simulink library "perturbations"  (R2025b)
settings: Solver=VariableStepAuto  StartTime=0.0  StopTime=10.0  RelTol=1e-3
values from neighbouring files (symbols this model uses):
  e_sun = deg2rad(23.45)    [project_review.m]
  I = diag([ix iy iz])    [project_review.m]
  j = [0.01; 0.05; 0.01;]    [project_review.m]
  mu_E = G_E*M_E    (= 398199)    [project_review.m]
  n_sun = 2*pi / T_sun    (= 1.99102127766e-07)    [project_review.m]
  R_E = 6378    [project_review.m]
  sim_step = 0.01    [project_review.m]
  w_E = 7.27 * 10^-5    (= 7.27e-05)    [project_review.m]
undefined symbols (not defined in the file or in its folder): area, g_10, g_11, h_11, N_B, P, r_Fi, r_sun, rho_d, rho_s
libraries: matrix_library x4, vec_norm x3
settings Model: Creator=nicol  LastModifiedBy=nicol

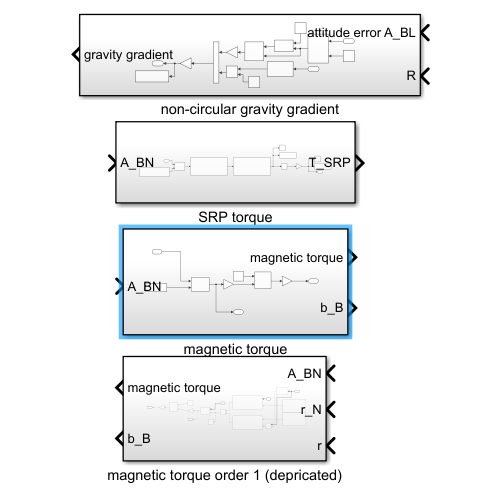
[thumbnail: Simulink's stored preview of the top-level diagram]
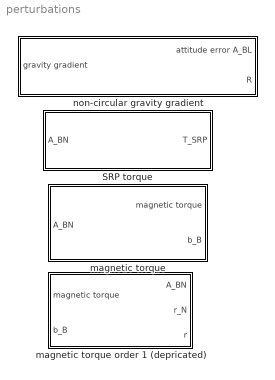
== system perturbations ==
  SRP torque : Subsystem
  magnetic torque : Subsystem
  magnetic torque order 1 (depricated) : Subsystem
  non-circular gravity gradient : Subsystem
      settings: PortSchema="{\"entries\":[{\"content\":{\"sides\":[{\"content\":{\"connectorIds\":[\"Out1\"]},\"type\":\"ConnectorPlacement.EquallySpacedRectSide\",\"uuid\":\"2a67419a-68c9-4369-a698-e6ac26417455\"},{\"content\":{\"connectorIds\":[\"In1\",\"In2\"],\"side\":\"RIGHT\"},\"type\":\"ConnectorPlacement.EquallySpacedRectSide\",\"uuid\":\"5f3f4c4a-6b79-4b92-8f4c-19ffa36753b2\"},{\"content\":{\"side\":\"TOP\"},\"type\":\"ConnectorPlacement.EquallySpacedRectSide\",\"uuid\":\"22c946b7-ea77-4444-a63c-d5b3d585f671\"}]},\"type\":\"ConnectorPlacement.EquallySpacedConnector\",\"uuid\":\"037c4a72-b28b-418e-a921-9da68dc0cd93\"}],\"packageUris\":[\"http://schema.mathworks.com/mf0/Connector/R2020b\"],\"version\":\"1.0\"}"

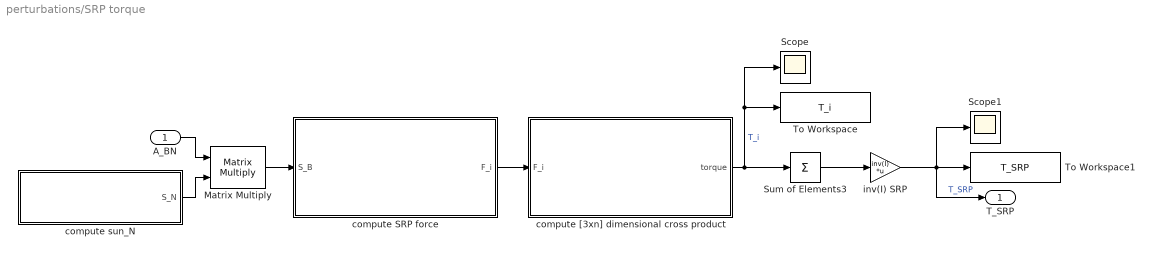
== system perturbations/SRP torque ==
  A_BN : Inport
  Matrix Multiply : Product  Multiplication=Matrix(*)
  Scope : Scope
      settings: ActiveDisplayYMinimum=-1  ActiveDisplayYMaximum=1  DataLoggingVariableName=ScopeData6
  Scope1 : Scope
      settings: ActiveDisplayYMinimum=-7.5910805781117744E-24  ActiveDisplayYMaximum=7.5910805781117744E-24  DataLoggingVariableName=ScopeData7
  Sum of Elements3 : Sum  Inputs=+  CollapseMode=Specified dimension  CollapseDim=2
  To Workspace : ToWorkspace  VariableName=T_i  SaveFormat=Timeseries  SampleTime=-1
  To Workspace1 : ToWorkspace  VariableName=T_SRP  SaveFormat=Timeseries  SampleTime=-1
  compute SRP force : Subsystem
  compute [3xn] dimensional cross product : Subsystem
  compute sun_N : Subsystem
  inv(I) SRP : Gain  Gain=inv(I)  Multiplication=Matrix(K*u)
  T_SRP : Outport
  wires:
  compute [3xn] dimensional cross product/1(torque) -> To Workspace/1, Scope/1, Sum of Elements3/1  "T_i"
  compute SRP force/1(F_i) -> compute [3xn] dimensional cross product/1(F_i)
  Matrix Multiply/1 -> compute SRP force/1(S_B)
  compute sun_N/1(S_N) -> Matrix Multiply/2
  inv(I) SRP/1 -> Scope1/1, T_SRP/1, To Workspace1/1  "T_SRP"
  A_BN/1 -> Matrix Multiply/1
  Sum of Elements3/1 -> inv(I) SRP/1

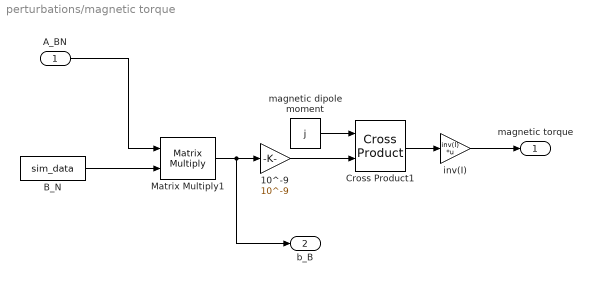
== system perturbations/magnetic torque ==
  A_BN : Inport
  10^-9 : Gain  Gain=10^-9
  B_N : FromWorkspace  VariableName=sim_data  SampleTime=sim_step  Interpolate=off  OutputAfterFinalValue=Holding final value
  Cross Product1 : matrix_library/Cross Product
  Matrix Multiply1 : Product  Multiplication=Matrix(*)
  inv(I) : Gain  Gain=inv(I)  Multiplication=Matrix(K*u)
  magnetic dipole moment : Constant  Value=j
  magnetic torque : Outport
  b_B : Outport  Port=2
  wires:
  A_BN/1 -> Matrix Multiply1/1
  magnetic dipole moment/1 -> Cross Product1/1
  B_N/1 -> Matrix Multiply1/2
  Cross Product1/1 -> inv(I)/1
  inv(I)/1 -> magnetic torque/1
  Matrix Multiply1/1 -> b_B/1, 10^-9/1
  10^-9/1 -> Cross Product1/2

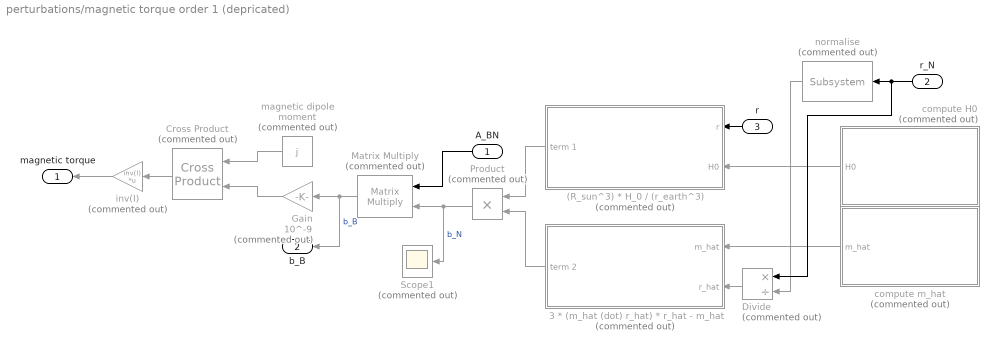
== system perturbations/magnetic torque order 1 (depricated) ==
  A_BN : Inport
  r_N : Inport  Port=2
  r : Inport  Port=3
  (R_sun^3) * H_0 / (r_earth^3) : Subsystem  Commented=on
      settings: PortSchema="{\"entries\":[{\"content\":{\"sides\":[{\"content\":{\"connectorIds\":[\"Out1\"]},\"type\":\"ConnectorPlacement.EquallySpacedRectSide\",\"uuid\":\"bbe988fc-17c4-4719-9870-44bc4a4e76ce\"},{\"content\":{\"connectorIds\":[\"In1\",\"In2\"],\"side\":\"RIGHT\"},\"type\":\"ConnectorPlacement.EquallySpacedRectSide\",\"uuid\":\"575c26dc-e0b7-4e24-b262-40ca05ffcfe5\"},{\"content\":{\"side\":\"TOP\"},\"type\":\"ConnectorPlacement.EquallySpacedRectSide\",\"uuid\":\"0bdf66e4-cddb-4706-9c0a-b23684b15a0a\"}]},\"type\":\"ConnectorPlacement.EquallySpacedConnector\",\"uuid\":\"a70c04a6-2589-454e-b011-fc54f6acc766\"}],\"packageUris\":[\"http://schema.mathworks.com/mf0/Connector/R2020b\"],\"version\":\"1.0\"}"
  3 * (m_hat (dot) r_hat) * r_hat - m_hat : Subsystem  Commented=on
  Cross Product : matrix_library/Cross Product  Commented=on
  Divide : Product  Commented=on  Inputs=*/
  Gain : Gain  Commented=on  Gain=10^-9
  Matrix Multiply : Product  Commented=on  Multiplication=Matrix(*)
  Product : Product  Commented=on
  Scope1 : Scope  Commented=on
      settings: DataLoggingVariableName=ScopeData2
  compute H0 : Subsystem  Commented=on
      settings: PortSchema="{\"entries\":[{\"content\":{\"sides\":[{\"content\":{\"connectorIds\":[\"Out1\"]},\"type\":\"ConnectorPlacement.EquallySpacedRectSide\",\"uuid\":\"69538ac4-798d-499e-8a01-9dbb1ae91e13\"},{\"content\":{\"side\":\"RIGHT\"},\"type\":\"ConnectorPlacement.EquallySpacedRectSide\",\"uuid\":\"e472a16b-e756-43b0-a684-24a7beecf6b1\"},{\"content\":{\"side\":\"TOP\"},\"type\":\"ConnectorPlacement.EquallySpacedRectSide\",\"uuid\":\"c0da2b73-1d3e-4f5f-b1be-bce0e733f90d\"}]},\"type\":\"ConnectorPlacement.EquallySpacedConnector\",\"uuid\":\"edf54bcc-843b-4ee1-a337-02c9fdc591b1\"}],\"packageUris\":[\"http://schema.mathworks.com/mf0/Connector/R2020b\"],\"version\":\"1.0\"}"
  compute m_hat : Subsystem  Commented=on
      settings: PortSchema="{\"entries\":[{\"content\":{\"sides\":[{\"content\":{\"connectorIds\":[\"Out1\"]},\"type\":\"ConnectorPlacement.EquallySpacedRectSide\",\"uuid\":\"69538ac4-798d-499e-8a01-9dbb1ae91e13\"},{\"content\":{\"side\":\"RIGHT\"},\"type\":\"ConnectorPlacement.EquallySpacedRectSide\",\"uuid\":\"e472a16b-e756-43b0-a684-24a7beecf6b1\"},{\"content\":{\"side\":\"TOP\"},\"type\":\"ConnectorPlacement.EquallySpacedRectSide\",\"uuid\":\"c0da2b73-1d3e-4f5f-b1be-bce0e733f90d\"}]},\"type\":\"ConnectorPlacement.EquallySpacedConnector\",\"uuid\":\"edf54bcc-843b-4ee1-a337-02c9fdc591b1\"}],\"packageUris\":[\"http://schema.mathworks.com/mf0/Connector/R2020b\"],\"version\":\"1.0\"}"
  inv(I) : Gain  Commented=on  Gain=inv(I)  Multiplication=Matrix(K*u)
  magnetic dipole moment : Constant  Commented=on  Value=j
  normalise : vec_norm/Subsystem  Commented=on  SystemSampleTime=-1  VariantActivationTime=update diagram  EmptyChoice=off  PassThrough=off  PassThroughVariantControl=(default)  EmptyChoiceVariantControl=(default)  AllowFlexibleInterface=on  Latency=0  AutoFrameSizeCalculation=off
  magnetic torque : Outport
  b_B : Outport  Port=2
  wires:
  A_BN/1 -> Matrix Multiply/1
  inv(I)/1 -> magnetic torque/1
  3 * (m_hat (dot) r_hat) * r_hat - m_hat/1(term 2) -> Product/2
  (R_sun^3) * H_0 / (r_earth^3)/1(term 1) -> Product/1
  compute m_hat/1(m_hat) -> 3 * (m_hat (dot) r_hat) * r_hat - m_hat/1(m_hat)
  magnetic dipole moment/1 -> Cross Product/1
  Product/1 -> Scope1/1, Matrix Multiply/2  "b_N"
  Matrix Multiply/1 -> b_B/1, Gain/1  "b_B"
  compute H0/1(H0) -> (R_sun^3) * H_0 / (r_earth^3)/2(H0)
  Divide/1 -> 3 * (m_hat (dot) r_hat) * r_hat - m_hat/2(r_hat)
  normalise/1 -> Divide/2
  r_N/1 -> normalise/1, Divide/1
  Cross Product/1 -> inv(I)/1
  Gain/1 -> Cross Product/2
  r/1 -> (R_sun^3) * H_0 / (r_earth^3)/1(r)

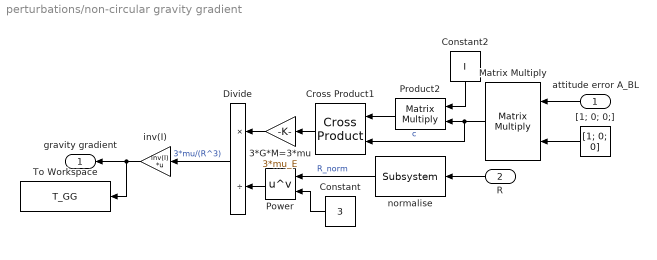
== system perturbations/non-circular gravity gradient ==
  attitude error A_BL : Inport
  R : Inport  Port=2
  3*G*M=3*mu : Gain  Gain=3*mu_E
  Constant : Constant  Value=3
  Constant2 : Constant  Value=I
  Cross Product1 : matrix_library/Cross Product
  Divide : Product  Inputs=*/
  Matrix Multiply : Product  Multiplication=Matrix(*)
  Power : Math  Operator=pow
  Product2 : Product  Multiplication=Matrix(*)
  To Workspace : ToWorkspace  VariableName=T_GG  SaveFormat=Timeseries  SampleTime=-1
  "[1; 0; 0;]" : Constant  Value=[1; 0; 0]
  inv(I) : Gain  Gain=inv(I)  Multiplication=Matrix(K*u)
  normalise : vec_norm/Subsystem  SystemSampleTime=-1  VariantActivationTime=update diagram  EmptyChoice=off  PassThrough=off  PassThroughVariantControl=(default)  EmptyChoiceVariantControl=(default)  AllowFlexibleInterface=on  Latency=0  AutoFrameSizeCalculation=off
  gravity gradient : Outport
  wires:
  normalise/1 -> Power/1  "R_norm"
  Power/1 -> Divide/2
  Constant/1 -> Power/2
  R/1 -> normalise/1
  inv(I)/1 -> To Workspace/1, gravity gradient/1
  3*G*M=3*mu/1 -> Divide/1
  "[1; 0; 0;]"/1 -> Matrix Multiply/2
  Product2/1 -> Cross Product1/1
  Cross Product1/1 -> 3*G*M=3*mu/1
  Constant2/1 -> Product2/1
  attitude error A_BL/1 -> Matrix Multiply/1
  Matrix Multiply/1 -> Product2/2, Cross Product1/2  "c"
  Divide/1 -> inv(I)/1  "3*mu/(R^3)"

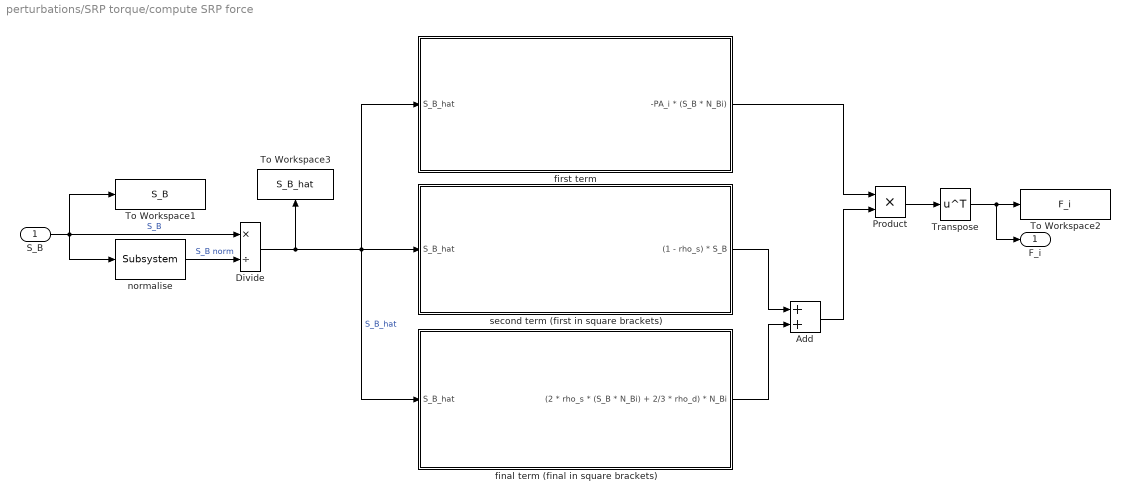
== system perturbations/SRP torque/compute SRP force ==
  S_B : Inport
  Add : Sum
  Divide : Product  Inputs=*/
  Product : Product
  To Workspace1 : ToWorkspace  VariableName=S_B  SaveFormat=Timeseries  SampleTime=-1
  To Workspace2 : ToWorkspace  VariableName=F_i  SaveFormat=Timeseries  SampleTime=-1
  To Workspace3 : ToWorkspace  VariableName=S_B_hat  SaveFormat=Timeseries  SampleTime=-1
  Transpose : Math  Operator=transpose
  final term (final in square brackets) : Subsystem
  first term : Subsystem
  normalise : vec_norm/Subsystem  SystemSampleTime=-1  VariantActivationTime=update diagram  EmptyChoice=off  PassThrough=off  PassThroughVariantControl=(default)  EmptyChoiceVariantControl=(default)  AllowFlexibleInterface=on  Latency=0  AutoFrameSizeCalculation=off
  second term (first in square brackets) : Subsystem
  F_i : Outport
  wires:
  final term (final in square brackets)/1((2 * rho_s * (S_B * N_Bi) + 2/3 * rho_d) * N_Bi) -> Add/2
  Transpose/1 -> F_i/1, To Workspace2/1
  first term/1(-PA_i * (S_B * N_Bi)) -> Product/1
  Add/1 -> Product/2
  second term (first in square brackets)/1((1 - rho_s) * S_B) -> Add/1
  Product/1 -> Transpose/1
  normalise/1 -> Divide/2  "S_B norm"
  Divide/1 -> second term (first in square brackets)/1(S_B_hat), first term/1(S_B_hat), final term (final in square brackets)/1(S_B_hat), To Workspace3/1  "S_B_hat"
  S_B/1 -> normalise/1, Divide/1, To Workspace1/1  "S_B"

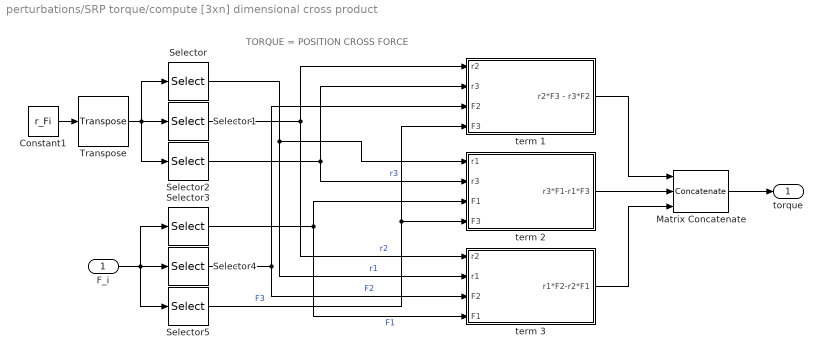
== system perturbations/SRP torque/compute [3xn] dimensional cross product ==
  note: TORQUE = POSITION CROSS FORCE
  F_i : Inport
  Constant1 : Constant  Value=r_Fi
  Matrix Concatenate : Concatenate  NumInputs=3  Mode=Multidimensional array
  Selector : Selector  NumberOfDimensions=2  InputPortWidth=3  IndexOptions=Index vector (dialog),Select all  Indices=1,1  OutputSizes=1,1
  Selector1 : Selector  NumberOfDimensions=2  InputPortWidth=3  IndexOptions=Index vector (dialog),Select all  Indices=2,1  OutputSizes=1,1
  Selector2 : Selector  NumberOfDimensions=2  InputPortWidth=3  IndexOptions=Index vector (dialog),Select all  Indices=3,1  OutputSizes=1,1
  Selector3 : Selector  NumberOfDimensions=2  InputPortWidth=3  IndexOptions=Index vector (dialog),Select all  Indices=1,1  OutputSizes=1,1
  Selector4 : Selector  NumberOfDimensions=2  InputPortWidth=3  IndexOptions=Index vector (dialog),Select all  Indices=2,1  OutputSizes=1,1
  Selector5 : Selector  NumberOfDimensions=2  InputPortWidth=3  IndexOptions=Index vector (dialog),Select all  Indices=3,1  OutputSizes=1,1
  Transpose : matrix_library/Transpose
  term 1 : Subsystem
  term 2 : Subsystem
  term 3 : Subsystem
  torque : Outport
  wires:
  Constant1/1 -> Transpose/1
  F_i/1 -> Selector4/1, Selector3/1, Selector5/1
  term 2/1(r3*F1-r1*F3) -> Matrix Concatenate/2
  Selector1/1 -> term 1/1(r2), term 3/1(r2)  "r2"
  term 3/1(r1*F2-r2*F1) -> Matrix Concatenate/3
  term 1/1(r2*F3 - r3*F2) -> Matrix Concatenate/1
  Selector4/1 -> term 3/3(F2), term 1/3(F2)  "F2"
  Selector5/1 -> term 1/4(F3), term 2/4(F3)  "F3"
  Selector2/1 -> term 1/2(r3), term 2/2(r3)  "r3"
  Transpose/1 -> Selector1/1, Selector/1, Selector2/1
  Selector3/1 -> term 3/4(F1), term 2/3(F1)  "F1"
  Selector/1 -> term 3/2(r1), term 2/1(r1)  "r1"
  Matrix Concatenate/1 -> torque/1

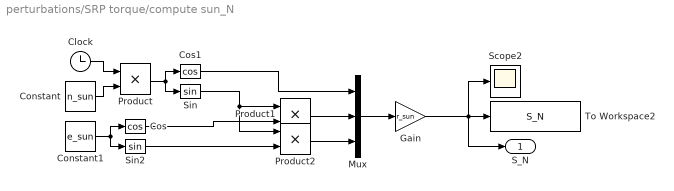
== system perturbations/SRP torque/compute sun_N ==
  Clock : Clock
  Constant : Constant  Value=n_sun
  Constant1 : Constant  Value=e_sun
  Cos : Trigonometry  Operator=cos
  Cos1 : Trigonometry  Operator=cos
  Gain : Gain  Gain=r_sun
  Mux : Mux  Inputs=3
  Product : Product
  Product1 : Product
  Product2 : Product
  Scope2 : Scope
      settings: ActiveDisplayYMinimum=-1.8699999999999996E+7  ActiveDisplayYMaximum=1.683E+8
  Sin : Trigonometry
  Sin2 : Trigonometry
  To Workspace2 : ToWorkspace  VariableName=S_N  SaveFormat=Timeseries  SampleTime=-1
  S_N : Outport
  wires:
  Constant1/1 -> Cos/1, Sin2/1
  Gain/1 -> S_N/1, To Workspace2/1, Scope2/1
  Cos1/1 -> Mux/1
  Product/1 -> Cos1/1, Sin/1
  Constant/1 -> Product/2
  Product1/1 -> Mux/2
  Product2/1 -> Mux/3
  Cos/1 -> Product1/2
  Sin/1 -> Product1/1, Product2/1
  Mux/1 -> Gain/1
  Sin2/1 -> Product2/2
  Clock/1 -> Product/1

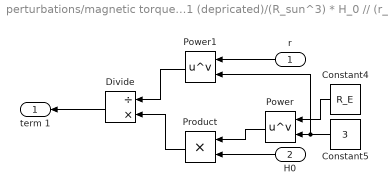
== system perturbations/magnetic torque order 1 (depricated)/(R_sun^3) * H_0 // (r_earth^3) ==
  r : Inport
  H0 : Inport  Port=2
  Constant4 : Constant  Value=R_E
  Constant5 : Constant  Value=3
  Divide : Product  Inputs=/*
  Power : Math  Operator=pow
  Power1 : Math  Operator=pow
  Product : Product
  term 1 : Outport
  wires:
  r/1 -> Power1/1
  Product/1 -> Divide/2
  H0/1 -> Product/2
  Divide/1 -> term 1/1
  Power1/1 -> Divide/1
  Constant5/1 -> Power1/2, Power/2
  Constant4/1 -> Power/1
  Power/1 -> Product/1

== system perturbations/magnetic torque order 1 (depricated)/3 * (m_hat (dot) r_hat) * r_hat - m_hat ==
  m_hat : Inport
  r_hat : Inport  Port=2
  Dot Product : DotProduct  OutDataTypeStr=Inherit: Inherit via internal rule
  Gain : Gain  Gain=3
  Product1 : Product
  Subtract : Sum  Inputs=-+
  term 2 : Outport
  wires:
  Gain/1 -> Subtract/2
  Product1/1 -> Gain/1
  Dot Product/1 -> Product1/1
  m_hat/1 -> Dot Product/1, Subtract/1
  Subtract/1 -> term 2/1
  r_hat/1 -> Dot Product/2, Product1/2

== system perturbations/magnetic torque order 1 (depricated)/compute H0 ==
  Add : Sum  Inputs=+++
  Constant1 : Constant  Value=g_10
  Constant2 : Constant  Value=g_11
  Constant3 : Constant  Value=h_11
  Square : Math  Operator=square
  Square Root : Sqrt
  Square1 : Math  Operator=square
  Square2 : Math  Operator=square
  H0 : Outport
  wires:
  Square/1 -> Add/1
  Square Root/1 -> H0/1
  Add/1 -> Square Root/1
  Square1/1 -> Add/2
  Square2/1 -> Add/3
  Constant3/1 -> Square2/1
  Constant1/1 -> Square/1
  Constant2/1 -> Square1/1

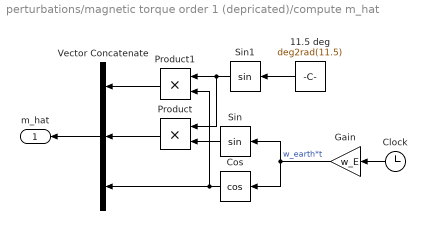
== system perturbations/magnetic torque order 1 (depricated)/compute m_hat ==
  11.5 deg : Constant  Value=deg2rad(11.5)
  Clock : Clock
  Cos : Trigonometry  Operator=cos
  Gain : Gain  Gain=w_E
  Product : Product
  Product1 : Product
  Sin : Trigonometry
  Sin1 : Trigonometry
  Vector Concatenate : Concatenate  NumInputs=3
  m_hat : Outport
  wires:
  Vector Concatenate/1 -> m_hat/1
  Sin/1 -> Product/2
  Clock/1 -> Gain/1
  Product/1 -> Vector Concatenate/2
  11.5 deg/1 -> Sin1/1
  Sin1/1 -> Product1/1, Product/1
  Gain/1 -> Sin/1, Cos/1  "w_earth*t"
  Cos/1 -> Vector Concatenate/3, Product1/2
  Product1/1 -> Vector Concatenate/1

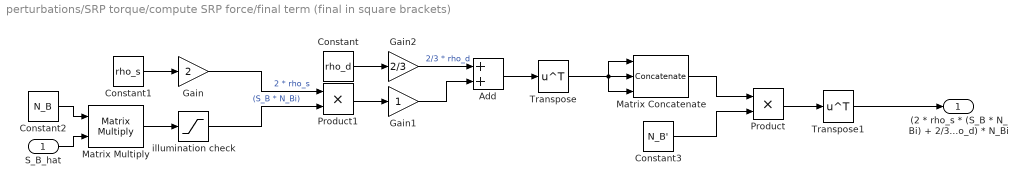
== system perturbations/SRP torque/compute SRP force/final term (final in square brackets) ==
  S_B_hat : Inport
  Add : Sum
  Constant : Constant  Value=rho_d
  Constant1 : Constant  Value=rho_s
  Constant2 : Constant  Value=N_B
  Constant3 : Constant  Value=N_B'
  Gain : Gain  Gain=2
  Gain1 : Gain
  Gain2 : Gain  Gain=2/3
  Matrix Concatenate : Concatenate  NumInputs=3  Mode=Multidimensional array
  Matrix Multiply : Product  Multiplication=Matrix(*)
  Product : Product
  Product1 : Product
  Transpose : Math  Operator=transpose
  Transpose1 : Math  Operator=transpose
  illumination check : Saturate  UpperLimit=inf  LowerLimit=0
  (2 * rho_s * (S_B * N_Bi) + 2/3 * rho_d) * N_Bi : Outport
  wires:
  Constant1/1 -> Gain/1
  Product1/1 -> Gain1/1
  Gain1/1 -> Add/2
  Transpose1/1 -> (2 * rho_s * (S_B * N_Bi) + 2/3 * rho_d) * N_Bi/1
  Constant3/1 -> Product/2
  Transpose/1 -> Matrix Concatenate/3, Matrix Concatenate/1, Matrix Concatenate/2
  S_B_hat/1 -> Matrix Multiply/2
  Constant2/1 -> Matrix Multiply/1
  Matrix Multiply/1 -> illumination check/1
  Gain/1 -> Product1/1  "2 * rho_s"
  Constant/1 -> Gain2/1
  Gain2/1 -> Add/1  "2/3 * rho_d"
  Add/1 -> Transpose/1
  Matrix Concatenate/1 -> Product/1
  Product/1 -> Transpose1/1
  illumination check/1 -> Product1/2  "(S_B * N_Bi)"

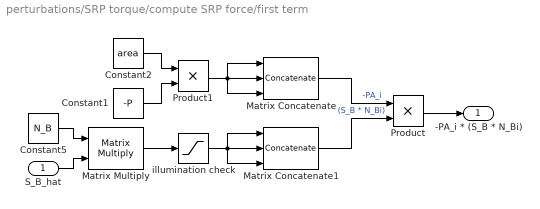
== system perturbations/SRP torque/compute SRP force/first term ==
  S_B_hat : Inport
  Constant1 : Constant  Value=-P
  Constant2 : Constant  Value=area
  Constant5 : Constant  Value=N_B
  Matrix Concatenate : Concatenate  NumInputs=3  Mode=Multidimensional array  ConcatenateDimension=2
  Matrix Concatenate1 : Concatenate  NumInputs=3  Mode=Multidimensional array  ConcatenateDimension=2
  Matrix Multiply : Product  Multiplication=Matrix(*)
  Product : Product
  Product1 : Product
  illumination check : Saturate  UpperLimit=inf  LowerLimit=0
  -PA_i * (S_B * N_Bi) : Outport
  wires:
  Product/1 -> -PA_i * (S_B * N_Bi)/1
  S_B_hat/1 -> Matrix Multiply/2
  Constant5/1 -> Matrix Multiply/1
  Constant2/1 -> Product1/1
  Constant1/1 -> Product1/2
  Product1/1 -> Matrix Concatenate/1, Matrix Concatenate/3, Matrix Concatenate/2
  Matrix Concatenate/1 -> Product/1  "-PA_i"
  illumination check/1 -> Matrix Concatenate1/3, Matrix Concatenate1/1, Matrix Concatenate1/2
  Matrix Concatenate1/1 -> Product/2  "(S_B * N_Bi)"
  Matrix Multiply/1 -> illumination check/1

== system perturbations/SRP torque/compute SRP force/second term (first in square brackets) ==
  S_B_hat : Inport
  Constant1 : Constant
  Constant2 : Constant  Value=rho_s
  Matrix Multiply : Product  Multiplication=Matrix(*)
  Subtract : Sum  Inputs=+-
  Transpose : Math  Operator=transpose
  (1 - rho_s) * S_B : Outport
  wires:
  Constant2/1 -> Subtract/2
  Constant1/1 -> Subtract/1
  Matrix Multiply/1 -> (1 - rho_s) * S_B/1
  Subtract/1 -> Matrix Multiply/1
  S_B_hat/1 -> Transpose/1
  Transpose/1 -> Matrix Multiply/2

== system perturbations/SRP torque/compute [3xn] dimensional cross product/term 1 ==
  r2 : Inport
  r3 : Inport  Port=2
  F2 : Inport  Port=3
  F3 : Inport  Port=4
  Product : Product
  Product1 : Product
  Subtract : Sum  Inputs=+-
  r2*F3 - r3*F2 : Outport
  wires:
  F3/1 -> Product/2
  Product/1 -> Subtract/1
  F2/1 -> Product1/2
  r2/1 -> Product/1
  Product1/1 -> Subtract/2
  Subtract/1 -> r2*F3 - r3*F2/1
  r3/1 -> Product1/1

== system perturbations/SRP torque/compute [3xn] dimensional cross product/term 2 ==
  r1 : Inport
  r3 : Inport  Port=2
  F1 : Inport  Port=3
  F3 : Inport  Port=4
  Product : Product
  Product1 : Product
  Subtract : Sum  Inputs=+-
  r3*F1-r1*F3 : Outport
  wires:
  F3/1 -> Product1/2
  Product1/1 -> Subtract/2
  Product/1 -> Subtract/1
  F1/1 -> Product/2
  r3/1 -> Product/1
  Subtract/1 -> r3*F1-r1*F3/1
  r1/1 -> Product1/1

== system perturbations/SRP torque/compute [3xn] dimensional cross product/term 3 ==
  r2 : Inport
  r1 : Inport  Port=2
  F2 : Inport  Port=3
  F1 : Inport  Port=4
  Product : Product
  Product1 : Product
  Subtract : Sum  Inputs=+-
  r1*F2-r2*F1 : Outport
  wires:
  F1/1 -> Product1/2
  r1/1 -> Product/1
  Product1/1 -> Subtract/2
  F2/1 -> Product/2
  Product/1 -> Subtract/1
  r2/1 -> Product1/1
  Subtract/1 -> r1*F2-r2*F1/1
